simulink model "showVolZcr"  (Simulink 7.5)
settings: Solver=ode45  StartTime=0.0  StopTime=inf  RelTol=1e-3
undefined symbols (not defined in the file or in its folder): get
libraries: dspmtrx3 x2, dspwin32 x1, dspbuff3 x1, dspsnks4 x1, dspstat3 x1
settings Model: Creator=jang  LastModifiedBy=jang
settings DataIOCC: SignalLoggingName=sigsOut
settings DebuggingCC: SaveWithParameterizedLinksMsg=none  SignalResolutionControl=TryResolveAllWithWarning  SolverPrmCheckMsg=none  MultiTaskDSMMsg=warning  MultiTaskCondExecSysMsg=none  StrictBusMsg=None
settings HardwareCC: TargetUnknown=on
settings RTWCC: IncludeERTFirstTime=on

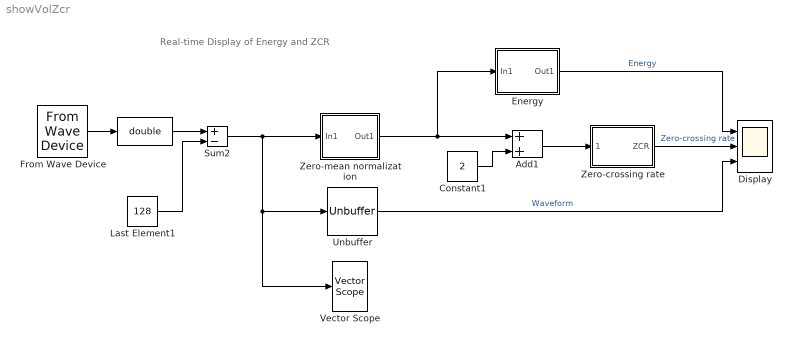
== system showVolZcr ==
  note: Real-time Display of Energy and ZCR
  " " : DataTypeConversion  OutDataTypeMode=double  OutDataTypeStr=double  SaturateOnIntegerOverflow=on  RndMeth=Zero
  Add1 : Sum  OutDataType=fixdt(1, 16)  OutScaling=2^-10
  Constant1 : Constant  Value=2  OutDataType=fixdt(1, 16)  OutScaling=2^0
  Display : Scope  NumInputPorts=3
      settings: TimeRange=10  YMin=-100~0~-128  YMax=200~100~127  DataFormat=Structure  SampleTime=0.1
  Energy : Subsystem
      mask Type: Compute energy of the input vector
      mask Display: disp('Energy')
  From Wave Device : dspwin32/From Wave Device  SampleRate=8000  UserRate=16000  SampleWidth=8  Stereo=off  SamplesPerFrame=256  QueueDuration=3  useDefaultDevice=on  userDeviceID=<empty>  dType=uint8
  Last Element1 : Constant  Value=128  OutDataTypeMode=double  OutDataType=sfix(16)  OutScaling=2^0  OutDataTypeStr=double
  Sum2 : Sum  Inputs=+-  OutDataType=sfix(16)  OutScaling=2^0  SaturateOnIntegerOverflow=on  InputSameDT=on  OutDataTypeStr=Inherit: Same as first input
  Unbuffer : dspbuff3/Unbuffer  ic=0
  Vector Scope : dspsnks4/Vector Scope  DialogController=dspdialog.VectorScope  DialogControllerArgs=DataTag0  ScopeProperties=off  Domain=Time  HorizSpan=1  DisplayProperties=off  AxisGrid=on  Memory=off  FrameNumber=on  AxisLegend=off  AxisZoom=off  OpenScopeAtSimStart=on  OpenScopeImmediately=off  FigPos=get(0,'defaultfigureposition')  AxisProperties=on  XUnits=Hertz  XRange=[0...Fs/2]  InheritXIncr=on  XIncr=1  XLabel=Time  XLimit=Auto  XMin=0  XMax=1  XStart=0  YUnits=dB  YLabel=Amplitude  LineProperties=off  XAxisParamsVer=6.8
      settings: YMin=-150  YMax=150
  Zero-crossing rate : Subsystem  Description=Find Local Min
      mask Type: Zero-crossing rate
      mask Display: disp('ZCR')
  Zero-mean normalization : Subsystem
      mask Type: Zero-mean normalization
      mask Display: disp('Zero-mean')
  wires:
  From Wave Device/1 -> " "/1
  Energy/1(Out1) -> Display/1  "Energy"
  " "/1 -> Sum2/1
  Sum2/1 -> Unbuffer/1, Vector Scope/1, Zero-mean normalization/1(In1)
  Last Element1/1 -> Sum2/2
  Zero-mean normalization/1(Out1) -> Energy/1(In1), Add1/1
  Unbuffer/1 -> Display/3  "Waveform"
  Zero-crossing rate/1(ZCR) -> Display/2  "Zero-crossing rate"
  Constant1/1 -> Add1/2
  Add1/1 -> Zero-crossing rate/1(In1 (Input Vec))

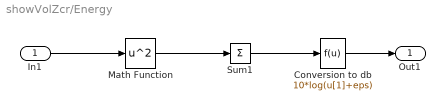
== system showVolZcr/Energy ==
  In1 : Inport  OutDataType=sfix(16)  OutScaling=2^0
  Conversion to db : Fcn  Expr=10*log(u[1]+eps)
  Math Function : Math  Operator=square  SaturateOnIntegerOverflow=on
  Sum1 : Sum  Inputs=+  OutDataType=sfix(16)  OutScaling=2^0  SaturateOnIntegerOverflow=on  InputSameDT=on  OutDataTypeStr=Inherit: Same as first input
  Out1 : Outport
  wires:
  Math Function/1 -> Sum1/1
  Sum1/1 -> Conversion to db/1
  In1/1 -> Math Function/1
  Conversion to db/1 -> Out1/1

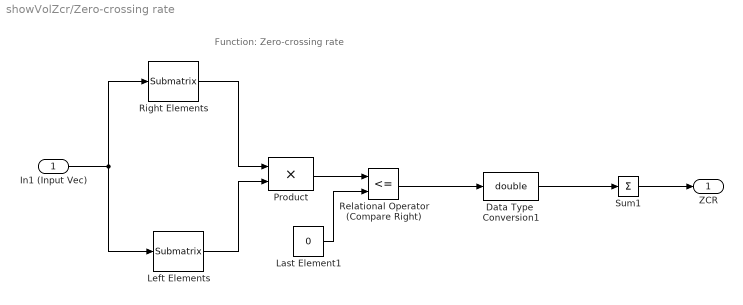
== system showVolZcr/Zero-crossing rate ==
  note: Function: Zero-crossing rate
  In1 (Input Vec) : Inport  OutDataType=sfix(16)  OutScaling=2^0
  Data Type  Conversion1 : DataTypeConversion  OutDataTypeMode=double  OutDataTypeStr=double  SaturateOnIntegerOverflow=on  RndMeth=Zero
  Last Element1 : Constant  Value=0  OutDataTypeMode=double  OutDataType=sfix(16)  OutScaling=2^0  OutDataTypeStr=double
  Left Elements : dspmtrx3/Submatrix  RowSpan=Range of rows  RowStartMode=Index  RowStartIndex=1  RowEndMode=Offset from last  RowEndIndex=1  ColSpan=All columns  ColStartMode=First  ColStartIndex=1  ColEndMode=Last  ColEndIndex=1
  Product : Product  OutDataType=sfix(16)  OutScaling=2^0  SaturateOnIntegerOverflow=on  OutDataTypeStr=Inherit: Same as first input
  Relational Operator (Compare Right) : RelationalOperator  Operator=<=  LogicOutDataTypeMode=boolean  OutDataTypeStr=boolean  InputSameDT=on
  Right Elements : dspmtrx3/Submatrix  RowSpan=Range of rows  RowStartMode=Index  RowStartIndex=2  RowEndMode=Last  RowEndIndex=1  ColSpan=All columns  ColStartMode=First  ColStartIndex=1  ColEndMode=Last  ColEndIndex=1
  Sum1 : Sum  Inputs=+  OutDataType=sfix(16)  OutScaling=2^0  SaturateOnIntegerOverflow=on  InputSameDT=on  OutDataTypeStr=Inherit: Same as first input
  ZCR : Outport
  wires:
  In1 (Input Vec)/1 -> Left Elements/1, Right Elements/1
  Right Elements/1 -> Product/1
  Left Elements/1 -> Product/2
  Sum1/1 -> ZCR/1
  Product/1 -> Relational Operator (Compare Right)/1
  Last Element1/1 -> Relational Operator (Compare Right)/2
  Relational Operator (Compare Right)/1 -> Data Type  Conversion1/1
  Data Type  Conversion1/1 -> Sum1/1

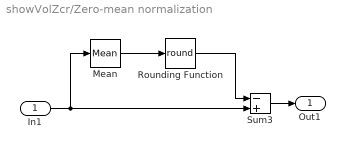
== system showVolZcr/Zero-mean normalization ==
  In1 : Inport  OutDataType=sfix(16)  OutScaling=2^0
  Mean : dspstat3/Mean  DialogController=dspDDGCreate  DialogControllerArgs=DataTag1  run=off  reset_popup=None  directionMode=Each column  dimension=1  treatSBRowAsCol=on  roiEnable=off  roiType=Rectangles  roiPortion=Entire ROI  roiOutput=Individual statistics for each ROI  roiFlag=off  outputDataTypeStr=Inherit: Same as accumulator  outputLastDataTypeStr=Inherit: Same as accumulator  outputMin=[]  outputMax=[]  roundingMode=Floor  overflowMode=off
  Rounding Function : Rounding  Operator=round
  Sum3 : Sum  Inputs=-+  OutDataType=sfix(16)  OutScaling=2^0  SaturateOnIntegerOverflow=on  InputSameDT=on  OutDataTypeStr=Inherit: Same as first input
  Out1 : Outport
  wires:
  Mean/1 -> Rounding Function/1
  Rounding Function/1 -> Sum3/1
  In1/1 -> Sum3/2, Mean/1
  Sum3/1 -> Out1/1
